simulink model "expanded"  (R2022b)
settings: Solver=VariableStepAuto  StartTime=0.0  StopTime=10.0  RelTol=1e-3
undefined symbols (not defined in the file or in its folder): sfunchk
libraries: truetime x3
settings Model: Creator=mona  LastModifiedBy=sunan
settings SolverCC: AlgebraicLoopSolver=TrustRegion
settings DataIOCC: ReturnWorkspaceOutputs=off
settings DebuggingCC: UnconnectedInputMsg=warning  UnconnectedOutputMsg=warning  UnconnectedLineMsg=warning  SFMachineParentedDataDiag=warning  ArithmeticOperatorsInVariantConditions=warning
settings ModelReferenceCC: EnableRefExpFcnMdlSchedulingChecks=on
settings SFSimCC: SimUseLocalCustomCode=off  CustomCodeUndefinedFunction=UseInterfaceOnly
settings RTWCC: RTWUseLocalCustomCode=off
settings CodeAppCC: StateflowObjectComments=on

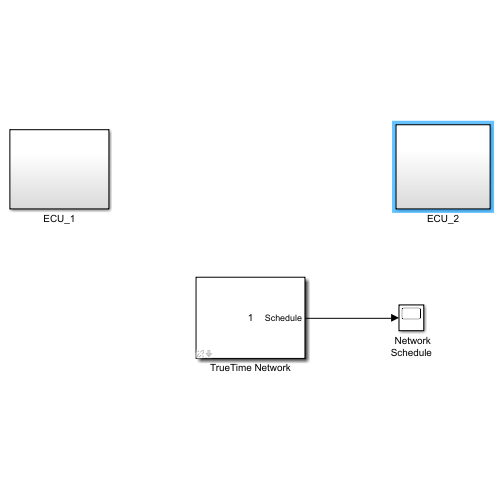
[thumbnail: Simulink's stored preview of the top-level diagram]
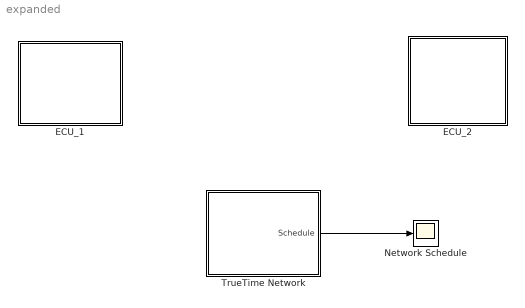
== system expanded ==
  " Network Schedule" : Scope
  ECU_1 : Subsystem
  ECU_2 : Subsystem
  TrueTime Network : Subsystem  AncestorBlock=truetime/TrueTime Network  mask(Real-Time Network){nwtype=CSMA/AMP (CAN), nwnbr=1, nnodes=6, rate=80000, minsize=80, lossprob=0, seed=0, bandwidths=[0.5 0.5], slotsize=512, schedule=[1 1 2], memsize=80000, buftype=Common buffer, overflow=Retransmit, dynSchedule=0, miniSlotSize=0, NIT=0, QSortMode=FIFO, sync=0, irtSchedule=0, nrtLength=0, nodeGraph=0, scheduleoutput=on}
      mask prompts: nwtype "Network type:"; nwnbr "Network number:"; nnodes "Number of nodes:"; rate "Data rate (bits/s):"; minsize "Minimum frame size (bits):"; lossprob "Loss probability (0-1):"; seed "Initial seed:"; bandwidths "Bandwidth allocations:"; slotsize "Slotsize (bits):"; schedule "Static schedule:"; memsize "Total switch memory (bits):"; buftype "Switch buffer type:"; overflow "Switch overflow behavior:"; dynSchedule "Dynamic Schedule:"; miniSlotSize "Mini slot size (bits):"; NIT "Network idle time (bits):"; QSortMode "Input Queue Sorted by:"; sync "Synchronization length (bits):"; irtSchedule "IRT Schedule [msgID from to start arrival]:"; nrtLength "RT Class 1/NRT length (bits):"; nodeGraph "Node connection graph (nbrOfnodes x nbrOfNodes):"; scheduleoutput "Show Schedule output port:"
      mask init:
      | ttnetwork_callback(gcb,nwnbr,nnodes,scheduleoutput)
      settings: LibrarySourceBlock=truetime/TrueTime Network
      mask TypeOptions nwtype: CSMA/CD (Ethernet) | CSMA/AMP (CAN) | Round Robin | FDMA | TDMA | Switched Ethernet | FlexRay | PROFINET | NCM
      mask Callback nwtype: ttnetwork_callback
      mask TypeOptions buftype: Common buffer | Symmetric output buffers
      mask TypeOptions overflow: Retransmit | Drop
      mask TypeOptions QSortMode: FIFO | Priority
      mask Display: disp(nwnbr)
  wires:
  TrueTime Network/1(Schedule) -> " Network Schedule"/1

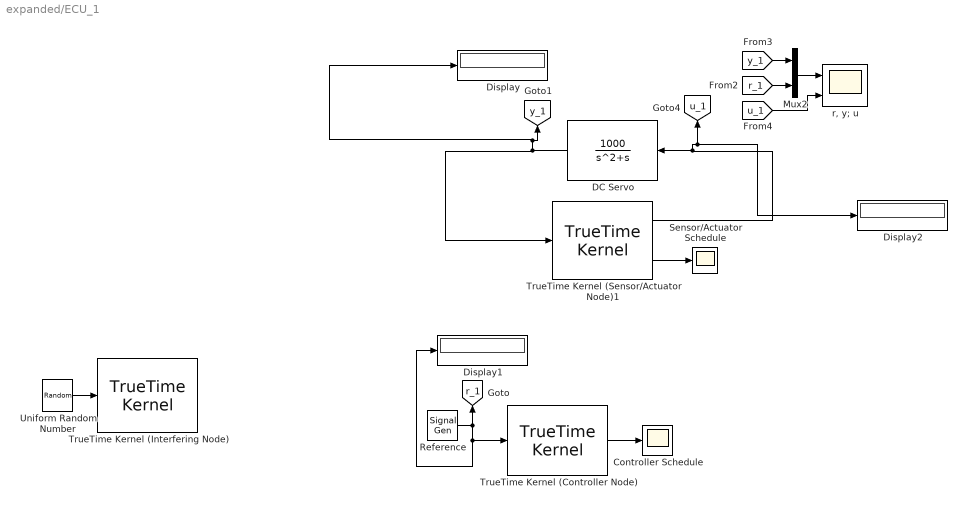
== system expanded/ECU_1 ==
  Controller Schedule : Scope
  DC Servo : TransferFcn  Numerator=1000  Denominator=[1 1 0]
  Display : Display
  Display1 : Display
  Display2 : Display
  Mux2 : Mux  Inputs=2
  Reference : SignalGenerator  WaveForm=square
  Sensor/Actuator Schedule : Scope
  TrueTime Kernel (Controller Node) : truetime/TrueTime Kernel  sfun=controller_init  args=0.0  ninputsoutputs=[1 0]  ntriggers=0  trigtype=rising  nwnodenbr=3  clockoffsetdrift=[0 0]  schedoutput=on  battery=off  poweroutput=off  label=1: 3
  TrueTime Kernel (Interfering Node) : truetime/TrueTime Kernel  sfun=interference_init  args=0.3  ninputsoutputs=[1 0]  ntriggers=0  trigtype=rising  nwnodenbr=1  clockoffsetdrift=[0 0]  schedoutput=off  battery=off  poweroutput=off  label=1: 1
  TrueTime Kernel (Sensor/Actuator Node)1 : truetime/TrueTime Kernel  sfun=sensor_actuator_init  args=[]  ninputsoutputs=[1 1]  ntriggers=0  trigtype=rising  nwnodenbr=2  clockoffsetdrift=[0 0]  schedoutput=on  battery=off  poweroutput=off  label=1: 2
  Uniform Random Number : UniformRandomNumber  Minimum=0  SampleTime=0.001
  "r, y; u" : Scope  NumInputPorts=2
  tag scope: r_1=global, u_1=global, y_1=global
  wires:
  [u_1] -> "r, y; u"/2
  TrueTime Kernel (Sensor/Actuator Node)1/1 -> DC Servo/1, Display2/1, [u_1]
  TrueTime Kernel (Sensor/Actuator Node)1/2 -> Sensor/Actuator Schedule/1
  DC Servo/1 -> Display/1, [y_1], TrueTime Kernel (Sensor/Actuator Node)1/1
  [y_1] -> Mux2/1
  [r_1] -> Mux2/2
  Mux2/1 -> "r, y; u"/1
  Reference/1 -> Display1/1, TrueTime Kernel (Controller Node)/1, [r_1]
  TrueTime Kernel (Controller Node)/1 -> Controller Schedule/1
  Uniform Random Number/1 -> TrueTime Kernel (Interfering Node)/1

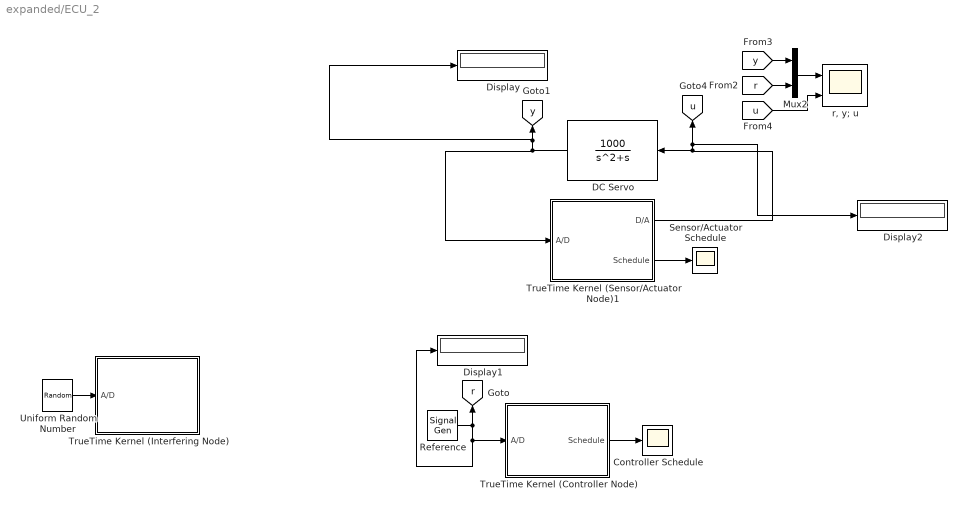
== system expanded/ECU_2 ==
  Controller Schedule : Scope
  DC Servo : TransferFcn  Numerator=1000  Denominator=[1 1 0]
  Display : Display
  Display1 : Display
  Display2 : Display
  Mux2 : Mux  Inputs=2
  Reference : SignalGenerator  WaveForm=square
  Sensor/Actuator Schedule : Scope
  TrueTime Kernel (Controller Node) : Subsystem  AncestorBlock=truetime/TrueTime Kernel  InitFcn=sfunchk(get_param(gcb,'sfun'));  mask{sfun=controller_init_1, args=0.0, ninputsoutputs=[1 0], ntriggers=0, trigtype=rising, nwnodenbr=6, clockoffsetdrift=[0 0], schedoutput=on, battery=off, poweroutput=off, label=1: 6}
      mask prompts: sfun "Name of init function (MEX or MATLAB):"; args "Init function argument (arbitrary struct):"; ninputsoutputs "Number of analog inputs and outputs:"; ntriggers "Number of external triggers:"; trigtype "Trigger type:"; nwnodenbr "(Network and) Node number(s):"; clockoffsetdrift "Local clock offset and drift:"; schedoutput "Show Schedule output port"; battery "Show Energy supply input port"; poweroutput "Show Power consumption output port"
      mask init:
      | ttkernel_callback(gcb,{sfun,args,ninputsoutputs,ntriggers,trigtype,nwnodenbr,clockoffsetdrift,schedoutput,battery,poweroutput})
      settings: LibrarySourceBlock=truetime/TrueTime Kernel  ErrorFcn=ttkernel_error
      mask TypeOptions trigtype: rising | falling | either
      mask Display: disp(get_param(gcb,'label'))
  TrueTime Kernel (Interfering Node) : Subsystem  AncestorBlock=truetime/TrueTime Kernel  InitFcn=sfunchk(get_param(gcb,'sfun'));  mask{sfun=interference_init_1, args=0.01, ninputsoutputs=[1 0], ntriggers=0, trigtype=rising, nwnodenbr=4, clockoffsetdrift=[0 0], schedoutput=off, battery=off, poweroutput=off, label=1: 4}
      mask prompts: sfun "Name of init function (MEX or MATLAB):"; args "Init function argument (arbitrary struct):"; ninputsoutputs "Number of analog inputs and outputs:"; ntriggers "Number of external triggers:"; trigtype "Trigger type:"; nwnodenbr "(Network and) Node number(s):"; clockoffsetdrift "Local clock offset and drift:"; schedoutput "Show Schedule output port"; battery "Show Energy supply input port"; poweroutput "Show Power consumption output port"
      mask init:
      | ttkernel_callback(gcb,{sfun,args,ninputsoutputs,ntriggers,trigtype,nwnodenbr,clockoffsetdrift,schedoutput,battery,poweroutput})
      settings: LibrarySourceBlock=truetime/TrueTime Kernel  ErrorFcn=ttkernel_error
      mask TypeOptions trigtype: rising | falling | either
      mask Display: disp(get_param(gcb,'label'))
  TrueTime Kernel (Sensor/Actuator Node)1 : Subsystem  AncestorBlock=truetime/TrueTime Kernel  InitFcn=sfunchk(get_param(gcb,'sfun'));  mask{sfun=sensor_actuator_init_1, args=[], ninputsoutputs=[1 1], ntriggers=0, trigtype=rising, nwnodenbr=5, clockoffsetdrift=[0 0], schedoutput=on, battery=off, poweroutput=off, label=1: 5}
      mask prompts: sfun "Name of init function (MEX or MATLAB):"; args "Init function argument (arbitrary struct):"; ninputsoutputs "Number of analog inputs and outputs:"; ntriggers "Number of external triggers:"; trigtype "Trigger type:"; nwnodenbr "(Network and) Node number(s):"; clockoffsetdrift "Local clock offset and drift:"; schedoutput "Show Schedule output port"; battery "Show Energy supply input port"; poweroutput "Show Power consumption output port"
      mask init:
      | ttkernel_callback(gcb,{sfun,args,ninputsoutputs,ntriggers,trigtype,nwnodenbr,clockoffsetdrift,schedoutput,battery,poweroutput})
      settings: LibrarySourceBlock=truetime/TrueTime Kernel  ErrorFcn=ttkernel_error
      mask TypeOptions trigtype: rising | falling | either
      mask Display: disp(get_param(gcb,'label'))
  Uniform Random Number : UniformRandomNumber  Minimum=0  SampleTime=0.001
  "r, y; u" : Scope  NumInputPorts=2
  tag scope: r=global, u=global, y=global
  wires:
  [u] -> "r, y; u"/2
  TrueTime Kernel (Sensor/Actuator Node)1/1(D/A) -> DC Servo/1, Display2/1, [u]
  TrueTime Kernel (Sensor/Actuator Node)1/2(Schedule) -> Sensor/Actuator Schedule/1
  DC Servo/1 -> Display/1, [y], TrueTime Kernel (Sensor/Actuator Node)1/1(A/D)
  [y] -> Mux2/1
  [r] -> Mux2/2
  Mux2/1 -> "r, y; u"/1
  Reference/1 -> Display1/1, TrueTime Kernel (Controller Node)/1(A/D), [r]
  TrueTime Kernel (Controller Node)/1(Schedule) -> Controller Schedule/1
  Uniform Random Number/1 -> TrueTime Kernel (Interfering Node)/1(A/D)

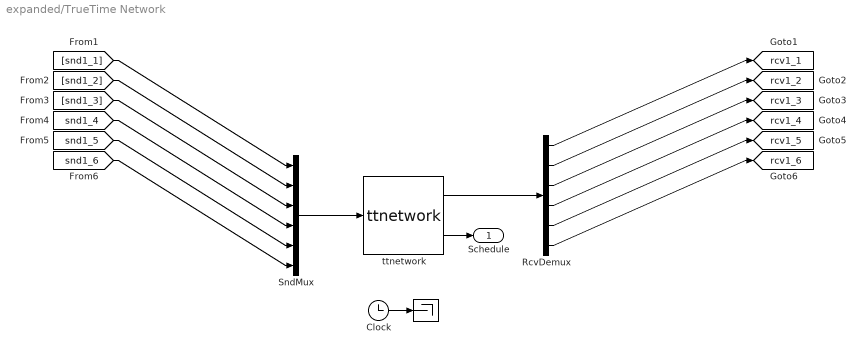
== system expanded/TrueTime Network ==
  " " : Terminator
  Clock : Clock
  RcvDemux : Demux  Outputs=6
      settings: DisplayOption=none
  SndMux : Mux  Inputs=6
  ttnetwork : S-Function  FunctionName=ttnetwork  Parameters=nwtype,nwnbr,nnodes,rate,minsize,lossprob,bandwidths,slotsize,schedule,memsize,buftype,overflow,seed,dynSchedule,miniSlotSize,NIT,QSortMode,sync,irtSchedule,nrtLength,nodeGraph  SFunctionDeploymentMode=off  EnableBusSupport=off
  Schedule : Outport
  tag scope: rcv1_1=global, rcv1_2=global, rcv1_3=global, rcv1_4=global, rcv1_5=global, rcv1_6=global
  wires:
  Clock/1 -> " "/1
  SndMux/1 -> ttnetwork/1
  ttnetwork/1 -> RcvDemux/1
  ttnetwork/2 -> Schedule/1
  [snd1_1] -> SndMux/1
  [snd1_2] -> SndMux/2
  [snd1_3] -> SndMux/3
  [snd1_4] -> SndMux/4
  [snd1_5] -> SndMux/5
  [snd1_6] -> SndMux/6
  RcvDemux/1 -> [rcv1_1]
  RcvDemux/2 -> [rcv1_2]
  RcvDemux/3 -> [rcv1_3]
  RcvDemux/4 -> [rcv1_4]
  RcvDemux/5 -> [rcv1_5]
  RcvDemux/6 -> [rcv1_6]

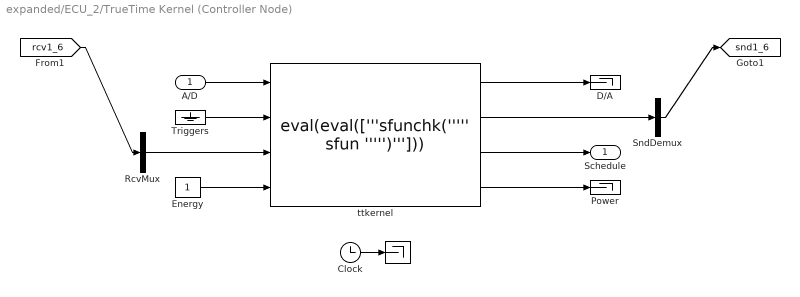
== system expanded/ECU_2/TrueTime Kernel (Controller Node) ==
  A/D : Inport
  " " : Terminator
  Clock : Clock
  D/A : Terminator
  Energy : Constant
  Power : Terminator
  RcvMux : Mux  Inputs=1
  SndDemux : Demux  Outputs=1
      settings: DisplayOption=none
  Triggers : Ground
  ttkernel : S-Function  FunctionName=eval(eval(['''sfunchk(''''' sfun ''''')''']))  Parameters=sfun, args, ninputsoutputs, ntriggers, trigtype, nwnodenbr, clockoffsetdrift  SFunctionDeploymentMode=off  EnableBusSupport=off
  Schedule : Outport
  tag scope: snd1_6=global
  wires:
  Clock/1 -> " "/1
  RcvMux/1 -> ttkernel/3
  Triggers/1 -> ttkernel/2
  ttkernel/3 -> Schedule/1
  ttkernel/1 -> D/A/1
  ttkernel/2 -> SndDemux/1
  A/D/1 -> ttkernel/1
  Energy/1 -> ttkernel/4
  ttkernel/4 -> Power/1
  [rcv1_6] -> RcvMux/1
  SndDemux/1 -> [snd1_6]

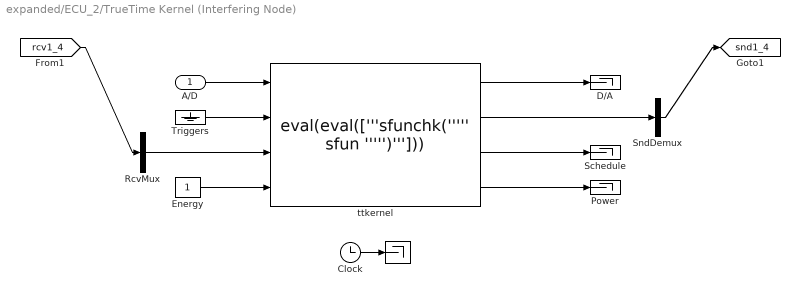
== system expanded/ECU_2/TrueTime Kernel (Interfering Node) ==
  A/D : Inport
  " " : Terminator
  Clock : Clock
  D/A : Terminator
  Energy : Constant
  Power : Terminator
  RcvMux : Mux  Inputs=1
  Schedule : Terminator
  SndDemux : Demux  Outputs=1
      settings: DisplayOption=none
  Triggers : Ground
  ttkernel : S-Function  FunctionName=eval(eval(['''sfunchk(''''' sfun ''''')''']))  Parameters=sfun, args, ninputsoutputs, ntriggers, trigtype, nwnodenbr, clockoffsetdrift  SFunctionDeploymentMode=off  EnableBusSupport=off
  tag scope: snd1_4=global
  wires:
  Clock/1 -> " "/1
  RcvMux/1 -> ttkernel/3
  Triggers/1 -> ttkernel/2
  ttkernel/3 -> Schedule/1
  ttkernel/1 -> D/A/1
  ttkernel/2 -> SndDemux/1
  A/D/1 -> ttkernel/1
  Energy/1 -> ttkernel/4
  ttkernel/4 -> Power/1
  [rcv1_4] -> RcvMux/1
  SndDemux/1 -> [snd1_4]

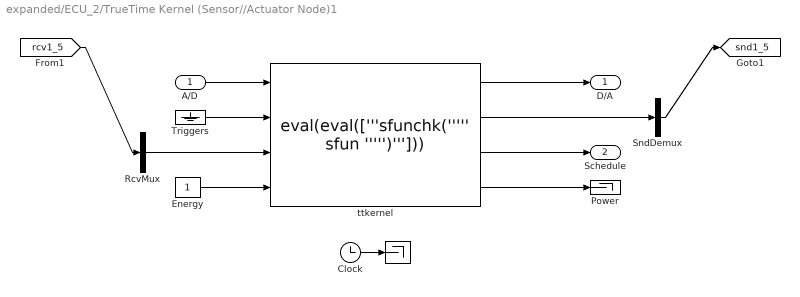
== system expanded/ECU_2/TrueTime Kernel (Sensor//Actuator Node)1 ==
  A/D : Inport
  " " : Terminator
  Clock : Clock
  Energy : Constant
  Power : Terminator
  RcvMux : Mux  Inputs=1
  SndDemux : Demux  Outputs=1
      settings: DisplayOption=none
  Triggers : Ground
  ttkernel : S-Function  FunctionName=eval(eval(['''sfunchk(''''' sfun ''''')''']))  Parameters=sfun, args, ninputsoutputs, ntriggers, trigtype, nwnodenbr, clockoffsetdrift  SFunctionDeploymentMode=off  EnableBusSupport=off
  D/A : Outport
  Schedule : Outport  Port=2
  tag scope: snd1_5=global
  wires:
  Clock/1 -> " "/1
  RcvMux/1 -> ttkernel/3
  Triggers/1 -> ttkernel/2
  ttkernel/3 -> Schedule/1
  ttkernel/1 -> D/A/1
  ttkernel/2 -> SndDemux/1
  A/D/1 -> ttkernel/1
  Energy/1 -> ttkernel/4
  ttkernel/4 -> Power/1
  [rcv1_5] -> RcvMux/1
  SndDemux/1 -> [snd1_5]
